simulink model "Hybrid_P2_Parallel"  (R2017b)
settings: Solver=FixedStepAuto  StartTime=0.0  StopTime=length(Speed)  FixedStep=0.01  MaxStep=0.01  RelTol=1e-3  EnableMultiTasking=on
PostLoadFcn:
  | , if any(exist('dsrtsu_mdlpostloadfcn', 'file') == [2, 3, 6]), try dsrtsu_mdlpostloadfcn('Execute', bdroot); catch fprintf('Error in PostLoadFcn (dsrtsu_mdlpostloadfcn) for model "%s":\n %s\n', bdroot, lasterr); end, end,
undefined symbols (not defined in the file): APP1_OOR, APP2_OOR, APP_Mismatch, Brk_Flt, cal, clt, Clutch, Clutch2, ClutchEngag, eng, Engine, EngOverTemp, ENGTRQ_MSMCH_Degraded_CP, ENGTRQ_MSMCH_ErrCritical_CP, ENGTRQ_MSMCH_LimpHome_CP, EngTrqMismatch, ess, ESSOverTemp, gb, KeyPos_Flt, LossCAN, MCUOverTemp, mot, MotDirMismatch, MotOverTemp, MotTrqMismatch, mph2kph, PRNDL_Flt, RegenFault, time, tloop
libraries: simulink x100, EC2_libraries x7, powerlib_meascontrol x2, lib_Actuators x1, CalculationGallon x1, lib_Chassis x1, autolibcoupling x1, autolibsharedcoupling x1, lib_DCDC x1, lib_Differential x1, lib_EMachine_2017a x1, lib_HVESS x1
(part 1 of 7)
settings Model: DSRTSU_INTERNAL_RTI_VER=480  DSRTSU_INTERNAL_RTI_TYPE=rti1006  RTICANMMDATA=struct('GeneralSetupData',struct('modelroot','D:\EcoCAR3\Controls\HIL\Y3\P2_Parallel_MIL_Model','generalsettings',struct('filesettings',struct('destfolder',struct('Name','RTICANMM_FILES','Check',1),'buildfolder',struct('Name','.','Check',1),'AbsDestfolder',struct('Name','D:\EcoCAR3\Controls\HIL\Y3\P2_Parallel_MIL_Model\RTICANMM_FILES'),'AbsBuildfolder',struct('Name','D:\EcoCAR3\Controls\HIL\Y3\P2_Parallel_MIL_Model'))),'options',struct('addpaths',1,'rmpaths',1,'addtrcexclusion',logical(1),'cannavigator',struct('checkmonitoring',0),'show_usrtrc',0,'use_usrtrc',0),'advanced',struct('options',[1 1 1 1 1 1 1 1 1 1 1 1 1 1 1 1 1 1 1 1 1 1 1 1 1 1 1 1 1 1 1 1 1 1 1 1 1 1 1 1 1 1 1 1 1 1 1 1 1 1 1 1 1 1 1 1 1 1 1 1 1 1 1 1 1 1 1 1 1 1 1 1 1 1 1 1 1 1 1 1 1 1 1 1 1 1 1 1 1 1 1 1 1 1 1 1 1 1 1 1]),'MPSetup',{{}},'modelname','P2_Parallel_MIL_02_16_2017','block','P2_Parallel_MIL_02_16_2017'))  DSRTSU_INTERNAL_RTIFPGA=70  SimulationMode=accelerator  Creator=EcoCar  LastModifiedBy=Lyu19
settings SolverCC: ExtrapolationOrder=1  NumberNewtonIterations=4
settings OptimizationCC: BlockReduction=off  OptimizeBlockIOStorage=off  BufferReuse=off  GlobalBufferReuse=off  ExpressionFolding=off  LocalBlockOutputs=off  EfficientMapNaN2IntZero=off
settings DebuggingCC: AllowSymbolicDim=off  NonBusSignalsTreatedAsBus=warning  SFUnexpectedBacktrackingDiag=warning  SFNoUnconditionalDefaultTransitionDiag=warning  SFExecutionAtInitializationDiag=none
settings HardwareCC: ProdBitPerPointer=32  ProdBitPerSizeT=32  ProdBitPerPtrDiffT=32  ProdLargestAtomicInteger=Integer  ProdWordSize=32  ProdHWDeviceType=Custom Processor->Custom  TargetBitPerPointer=64  TargetBitPerSizeT=64  TargetBitPerPtrDiffT=64  TargetLongLongMode=on  TargetIntDivRoundTo=Zero  TargetEndianess=LittleEndian  TargetWordSize=64  TargetHWDeviceType=MATLAB Host  ProdEqTarget=off
settings ModelReferenceCC: PropagateSignalLabelsOutOfModel=off
settings CodeAppCC: MaxIdLength=128  StateflowObjectComments=on
settings GRTTargetCC: TargetLangStandard=C89/C90 (ANSI)  CombineOutputUpdateFcns=off  GRTInterface=on
settings ConfigComp: CovMetricSettings=dw  CovHtmlReporting=on  CovSaveCumulativeToWorkspaceVar=on  CovSaveSingleToWorkspaceVar=on  CovExternalEMLEnable=off
settings SimscapeCC: SimscapeNormalizeSystem=off

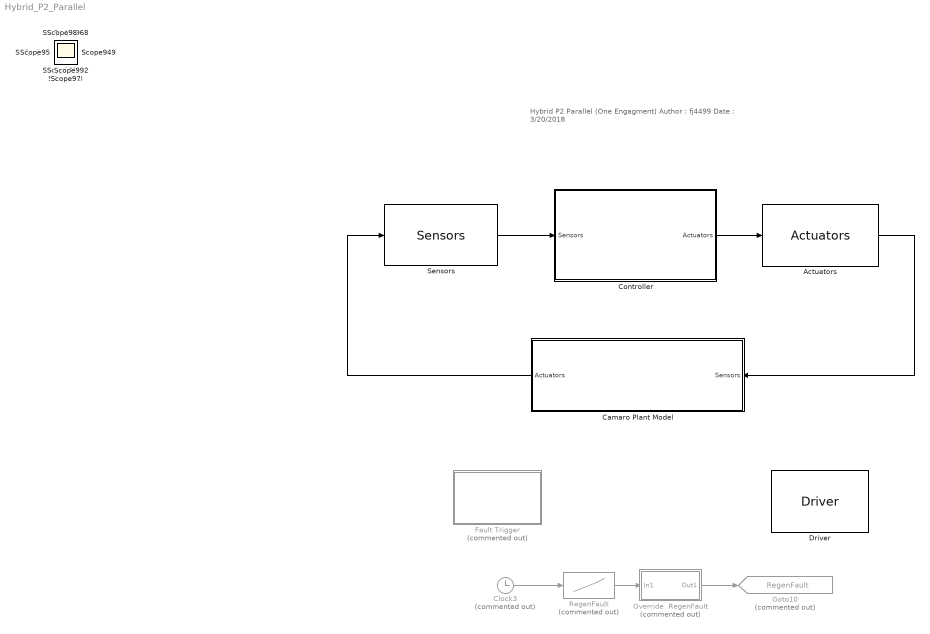
== system Hybrid_P2_Parallel ==
  note: Hybrid P2 Parallel (One Engagment)
      |
      | Author : fj4499
      | Date : 3/20/2018
  Actuators : lib_Actuators/Actuators
  Camaro Plant Model : Subsystem
      mask Display: image('Images/Vehicle.jpg')
  Clock3 : Clock  Commented=on
  Controller : Subsystem
      mask Display: image('Images/HCU.jpg')
  Driver : lib_Driver/Driver  SystemSampleTime=-1
  "Fault Trigger " : Subsystem  Commented=on  mask(Fault Trigger){Mismatch_APP_ON=on, APP1_OOR_ON=on, APP2_OOR_ON=on, Brk_Flt_ON=on, KeyPos_Flt_ON=on, PRNDL_Flt_ON=on, LossCAN_ON=on, MotTrqMismatch_ON=on, MotDirMismatch_ON=on, EngTrqMismatch_ON=on, MotOverTemp_ON=on, MCUOverTemp_ON=on, EngOverTemp_ON=on, ESSOverTemp_ON=on, ClutchEngagFlt=on}
      mask help:
      | Check the box: override the fault (Control Port value=1;)
      | Uncheck the box: Implement the fault (Control Port value=0;)
      mask DialogControl DriverInterfaceFault Prompt: Driver Interface Fault
      mask DialogControl Container3 Prompt: Component Fault
      mask Display:
      | plot([1 2 2.01 3 4], [0 0 1 1 1]);
      | disp('           Fault Trigger')
  Goto10 : Goto  Commented=on  GotoTag=RegenFault  TagVisibility=global
  Override  RegenFault : Subsystem  Commented=on
  RegenFault : Lookup  Commented=on  InputValues=time  Table=RegenFault  LookUpMeth=Interpolation-Use End Values  OutDataTypeStr=int8
  Sensors : lib_Sensors_2017a/Sensors
  Scope{,1..133} (134 alike) : Scope
  wires:
  Clock3/1 -> RegenFault/1
  RegenFault/1 -> Override  RegenFault/1(In1)
  Override  RegenFault/1(Out1) -> Goto10/1
  Controller/1(Actuators) -> Actuators/1
  Actuators/1 -> Camaro Plant Model/1(Sensors)
  Camaro Plant Model/1(Actuators) -> Sensors/1
  Sensors/1 -> Controller/1(Sensors)

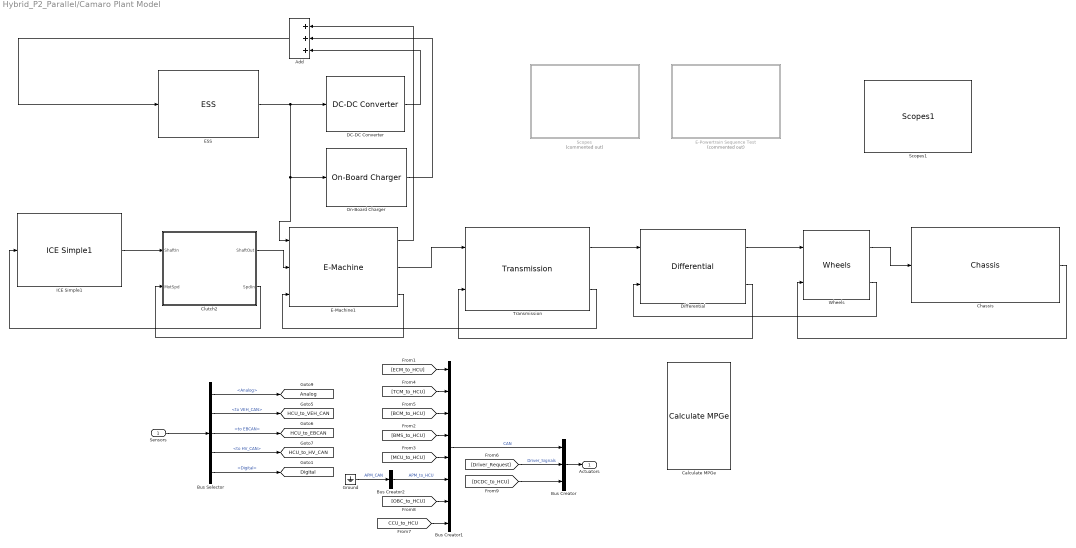
== system Hybrid_P2_Parallel/Camaro Plant Model ==
  Sensors : Inport
  Add : Sum  Inputs=+++
      mask Display:
      | port_label('input',1,'+');
      | port_label('input',2,'+');
      | port_label('input',3,'+');
  Bus Creator : BusCreator  Inputs=3
  Bus Creator1 : BusCreator  Inputs=8
  Bus Creator2 : BusCreator  Inputs=1
  Bus Selector : BusSelector  OutputSignals=Analog,CAN.to VEH_CAN,CAN.to EBCAN,CAN.to HV_CAN,Digital
  Calculate MPGe : CalculationGallon/Calculate MPGe
  Chassis : lib_Chassis/Chassis  SystemSampleTime=-1
  Clutch2 : Subsystem  AncestorBlock=Clutch/Clutch2
      mask Display:
      | image('Images/Clutch.jpg')
      | color('red');
      | port_label('Input',1,'ShaftIn');
      | port_label('Input',2,'SpdOut');
      | port_label('Output',1,'ShaftOut');
      | port_label('Output',2,'SpdIn');
  DC-DC Converter : lib_DCDC/DC-DC Converter  SystemSampleTime=-1
  Differential : lib_Differential/Differential  SystemSampleTime=-1
  E-Machine1 : lib_EMachine_2017a/E-Machine  SystemSampleTime=-1
  E-Powertrain Sequence Test : Subsystem  Commented=on
      mask Display: image('Images/Scope.jpg')
  ESS : lib_HVESS/ESS  SystemSampleTime=-1
  Ground : Ground
  ICE Simple1 : lib_Engine/ICE Simple1  SystemSampleTime=-1
  On-Board Charger : lib_OBC/On-Board Charger  SystemSampleTime=-1
      settings: SourceProductName=The database C:\Users\vrajm\AppData\Roaming\MathWorks\MATLAB\R2017b\slblocks_master.db is locked, or a table in the database is locked. (database is locked)
  Scopes : Subsystem  Commented=on
      mask Display: image('Images/Scope.jpg')
  Scopes1 : Scope_new/Scopes1  SystemSampleTime=-1
  Transmission : lib_Transmission/Transmission  SystemSampleTime=-1
  Wheels : lib_Wheels/Wheels  SystemSampleTime=-1
  Actuators : Outport
  tag scope: Analog=global, Digital=global, HCU_to_EBCAN=global, HCU_to_HV_CAN=global, HCU_to_VEH_CAN=global
  wires:
  Differential/1 -> Wheels/1
  Wheels/1 -> Chassis/1
  Chassis/1 -> Wheels/2
  Differential/2 -> Transmission/2
  Transmission/1 -> Differential/1
  ESS/1 -> E-Machine1/1, On-Board Charger/1, DC-DC Converter/1
  DC-DC Converter/1 -> Add/3
  On-Board Charger/1 -> Add/2
  Add/1 -> ESS/1
  Transmission/2 -> E-Machine1/3
  E-Machine1/2 -> Transmission/1
  E-Machine1/1 -> Add/1
  Bus Creator/1 -> Actuators/1
  Sensors/1 -> Bus Selector/1
  Bus Selector/1 -> [Analog]  "<Analog>"
  Bus Selector/2 -> [HCU_to_VEH_CAN]  "<to VEH_CAN>"
  Bus Selector/3 -> [HCU_to_EBCAN]  "<to EBCAN>"
  Bus Selector/4 -> [HCU_to_HV_CAN]  "<to HV_CAN>"
  Bus Selector/5 -> [Digital]  "<Digital>"
  Wheels/2 -> Differential/2
  E-Machine1/3 -> Clutch2/2(MotSpd)
  [ECM_to_HCU] -> Bus Creator1/1
  [TCM_to_HCU] -> Bus Creator1/2
  [BCM_to_HCU] -> Bus Creator1/3
  [BMS_to_HCU] -> Bus Creator1/4
  [MCU_to_HCU] -> Bus Creator1/5
  Bus Creator2/1 -> Bus Creator1/6  "APM_to_HCU"
  [OBC_to_HCU] -> Bus Creator1/7
  Bus Creator1/1 -> Bus Creator/1  "CAN"
  [Driver_Request] -> Bus Creator/2  "Driver_Signals"
  [DCDC_to_HCU] -> Bus Creator/3
  Ground/1 -> Bus Creator2/1  "APM_CAN"
  Clutch2/1(ShaftOut) -> E-Machine1/2
  Clutch2/2(SpdIn) -> ICE Simple1/1
  [CCU_to_HCU] -> Bus Creator1/8
  ICE Simple1/1 -> Clutch2/1(ShaftIn)

== system Hybrid_P2_Parallel/Controller ==
  Sensors : Inport
  HSC : Subsystem
  Actuators : Outport
  wires:
  HSC/1(Actuators) -> Actuators/1
  Sensors/1 -> HSC/1(Sensors)

== system Hybrid_P2_Parallel/Fault Trigger  ==
  Clock3 : Clock
  Component Diagnostics setting : Subsystem
  Driver Interface Diagnostics setting : Subsystem
  wires:
  Clock3/1 -> Component Diagnostics setting/1(time), Driver Interface Diagnostics setting/1(time)

== system Hybrid_P2_Parallel/Override  RegenFault ==
  note: This subsystem is used to override the model value of a signal to a constant value
  note: Override Switch Subsystem
  In1 : Inport
  Constant : Constant  Value=0
  Multiport Switch : MultiPortSwitch  DataPortOrder=Zero-based contiguous  Inputs=2
  Signal Override Switch 0 = Use Model 1 = Use Constant : Constant  Value=0
  Out1 : Outport
  wires:
  Signal Override Switch 0 = Use Model 1 = Use Constant/1 -> Multiport Switch/1
  In1/1 -> Multiport Switch/2
  Multiport Switch/1 -> Out1/1
  Constant/1 -> Multiport Switch/3

== system Hybrid_P2_Parallel/Camaro Plant Model/Clutch2 ==
  ShaftIn : Inport
  MotSpd : Inport  Port=2
  CCU : Subsystem
      mask Display: image('SoftECU.jpg')
  Clutch Plant : Subsystem
      mask Display:
      | image('Images/Clutch.jpg')
      | color('red');
      | port_label('Input',2,'ShaftIn');
      | port_label('Input',3,'SpdOut');
      | port_label('Output',3,'ShaftOut');
      | port_label('Output',2,'SpdIn');
  ShaftOut : Outport
  SpdIn : Outport  Port=2
  tag scope: CCU_to_HCU=global
  wires:
  Clutch Plant/1(Out1) -> CCU/2(Clutch Feedback)
  CCU/1("CCU_CAN ") -> [CCU_to_HCU]
  Clutch Plant/3(MotorShaft Out) -> ShaftOut/1
  Clutch Plant/2(Spdin) -> SpdIn/1
  MotSpd/1 -> Clutch Plant/3(SpdOut)
  ShaftIn/1 -> Clutch Plant/2(In2)
  CCU/2("Actuator command ") -> Clutch Plant/1(In1)
  [HCU_to_EBCAN] -> CCU/1(HSC Commands)

== system Hybrid_P2_Parallel/Camaro Plant Model/E-Powertrain Sequence Test ==
  Scope : Scope  NumInputPorts=4
  Terminator : Terminator
  wires:
  [KeyPosition] -> Scope/1  "Key Position"
  [InverterEnabled] -> Scope/2  "Inverter Enabled"
  [MO_BMS_Sollmodus] -> Scope/3  "Contactors Status"
  [DCDC_Status] -> Scope/4  "DCDC Status"
  [ShftLvrPos] -> Terminator/1  "Shift Lever Postion"

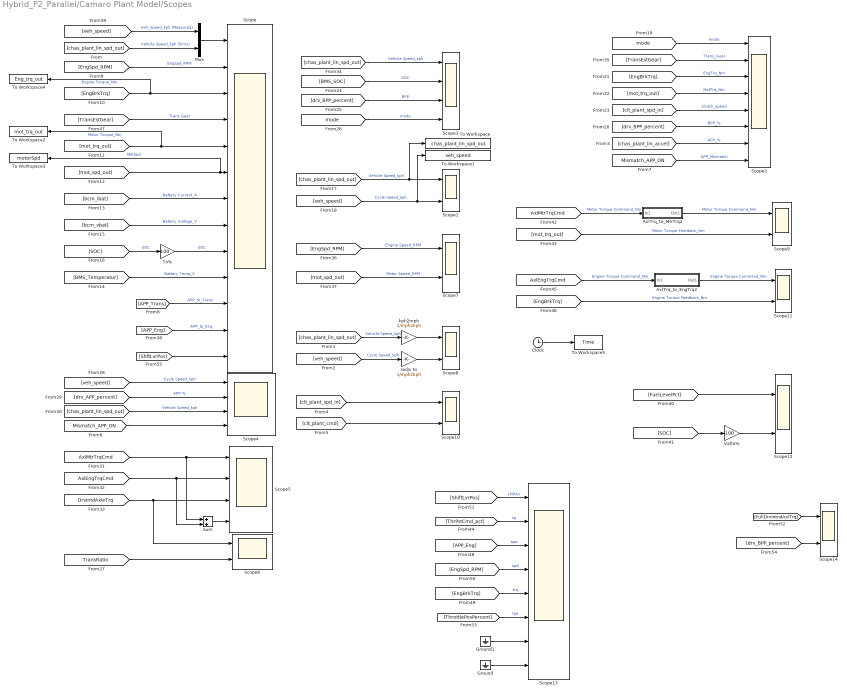
== system Hybrid_P2_Parallel/Camaro Plant Model/Scopes ==
  AxlTrq_to_EngTrq2 : Subsystem
  AxlTrq_to_MtrTrq2 : Subsystem
  Clock : Clock
      settings: Decimation=WORKSPACE_DECIMATION
  Ground : Ground
  Ground1 : Ground
  Mux : Mux  Inputs=2
  Scope : Scope  NumInputPorts=13
  Scope{1,6..12,14} (9 alike) : Scope  NumInputPorts=2
  Scope13 : Scope  NumInputPorts=8
  Scope2 : Scope  NumInputPorts=8
  Scope3 : Scope  NumInputPorts=4
  Scope4 : Scope  NumInputPorts=4
  Scope5 : Scope  NumInputPorts=4
  Sum : Sum
  To Workspace : ToWorkspace  VariableName=chas_plant_lin_spd_out  SampleTime=-1
  To Workspace1 : ToWorkspace  VariableName=veh_speed  SampleTime=-1
  To Workspace2 : ToWorkspace  VariableName=mot_trq_out  SampleTime=-1
  To Workspace3 : ToWorkspace  VariableName=motorSpd  SampleTime=-1
  To Workspace4 : ToWorkspace  VariableName=Eng_trq_out  SampleTime=-1
  To Workspace5 : ToWorkspace  VariableName=Time  SampleTime=-1
      settings: Decimation=WORKSPACE_DECIMATION
  To% : Gain  Gain=100
  Valto% : Gain  Gain=100
  kph2mph : Gain  Gain=1/mph2kph
  "rad/s to " : Gain  Gain=1/mph2kph
  wires:
  [chas_plant_lin_spd_out] -> Mux/2  "Vehicle Speed_kph (Simu)"
  [EngSpd_RPM] -> Scope/2  "EngSpd_RPM"
  [EngBrkTrq] -> To Workspace4/1, Scope/3  "Engine Torque_Nm"
  [mot_spd_out] -> To Workspace3/1, Scope/6  "MotSpd"
  [BMS_Temperatur] -> Scope/10  "Battery Temp_C"
  [mot_trq_out] -> To Workspace2/1, Scope/5  "Motor Torque_Nm"
  To%/1 -> Scope/9  "SOC"
  [TransEstGear] -> Scope/4  "Trans Gear"
  [bcm_ibat] -> Scope/7  "Battery Current_A"
  [chas_plant_lin_spd_out] -> Scope3/1  "Vehicle Speed_kph"
  [BMS_SOC] -> Scope3/2  "SOC"
  [drv_BPP_percent] -> Scope3/3  "BPP"
  [mode] -> Scope3/4  "mode"
  [chas_plant_lin_spd_out] -> To Workspace/1, Scope1/1  "Vehicle Speed_kph"
  [veh_speed] -> To Workspace1/1, Scope1/2  "Cycle Speed_kph"
  [mode] -> Scope2/1  "mode"
  [EngBrkTrq] -> Scope2/3  "EngTrq_Nm"
  [mot_trq_out] -> Scope2/4  "MotTrq_Nm"
  [clt_plant_spd_in] -> Scope2/5  "Clutch_speed"
  [EngSpd_RPM] -> Scope7/1  "Engine Speed_RPM"
  [mot_spd_out] -> Scope7/2  "Motor Speed_RPM"
  [veh_speed] -> Scope4/1  "Cycle Speed_kph"
  [drv_APP_percent] -> Scope4/2  "APP %"
  [chas_plant_lin_spd_out] -> Scope4/3  "Vehicle Speed_kph"
  [AxlMtrTrqCmd] -> Sum/1, Scope5/1
  [AxlEngTrqCmd] -> Sum/2, Scope5/2
  [DrvIntdAxleTrq] -> Scope6/1, Scope5/3
  Sum/1 -> Scope5/4
  [TransRatio] -> Scope6/2
  [AxlMtrTrqCmd] -> AxlTrq_to_MtrTrq2/1(In1)  "Motor Torque Command_Nm"
  [mot_trq_out] -> Scope9/2  "Motor Torque Feedback_Nm"
  [AxlEngTrqCmd] -> AxlTrq_to_EngTrq2/1(In1)  "Engine Torque Command_Nm"
  [EngBrkTrq] -> Scope11/2  "Engine Torque Feedback_Nm"
  [chas_plant_lin_spd_out] -> kph2mph/1  "Vehicle Speed_kph"
  [veh_speed] -> "rad/s to "/1  "Cycle Speed_kph"
  kph2mph/1 -> Scope8/1
  "rad/s to "/1 -> Scope8/2
  [TransEstGear] -> Scope2/2  "Trans_Gear"
  [drv_BPP_percent] -> Scope2/6  "BPP_%"
  [chas_plant_lin_accel] -> Scope2/7  "APP_%"
  AxlTrq_to_MtrTrq2/1(Out1) -> Scope9/1  "Motor Torque Command_Nm"
  AxlTrq_to_EngTrq2/1(Out1) -> Scope11/1  "Engine Torque Command_Nm"
  [bcm_vbat] -> Scope/8  "Battery Voltage_V"
  [clt_plant_spd_in] -> Scope10/1
  [clt_plant_cmd] -> Scope10/2
  [Mismatch_APP_ON] -> Scope4/4
  [Mismatch_APP_ON] -> Scope2/8  "APP_Mismatch"
  [SOC] -> To%/1  "SOC"
  [APP_Trans] -> Scope/11  "APP_to_Trans"
  [APP_Eng] -> Scope/12  "APP_to_Eng"
  Mux/1 -> Scope/1
  [veh_speed] -> Mux/1  "Veh_Speed_kph (Measured)"
  Clock/1 -> To Workspace5/1
  [FuelLevelPct] -> Scope12/1
  [SOC] -> Valto%/1
  Valto%/1 -> Scope12/2
  [ShiftLvrPos] -> Scope13/1  "shiftlvr"
  [ThrPstCmd_pct] -> Scope13/2  "tp"
  [APP_Eng] -> Scope13/3  "app"
  [EngSpd_RPM] -> Scope13/4  "spd"
  [EngBrkTrq] -> Scope13/5  "trq"
  [ThrottlePosPercent] -> Scope13/6  "tpp"
  Ground/1 -> Scope13/8
  Ground1/1 -> Scope13/7
  [FullDrvIntndAxlTrq] -> Scope14/1
  [drv_BPP_percent] -> Scope14/2
  [ShftLvrPos] -> Scope/13

== system Hybrid_P2_Parallel/Controller/HSC ==
  Sensors : Inport
  Camaro Fault Detection : Subsystem
  Driver_Requests : Subsystem  RequirementInfo={} %GIDa_7669cec5_5f7d_402f_871c_1fc3f99e6295
  Powertrain Manager : Subsystem
  Actuators : Outport
  wires:
  Driver_Requests/1(DriverRequests) -> Powertrain Manager/2(Driver Request)
  Camaro Fault Detection/1(Diagnostic) -> Driver_Requests/2("Diagnostic "), Powertrain Manager/3(Fault Detection)
  Powertrain Manager/1(Out1) -> Actuators/1
  Sensors/1 -> Driver_Requests/1(Sensors), Powertrain Manager/1(Sensors), Camaro Fault Detection/1(Sensors)
  Powertrain Manager/2(Controls) -> Driver_Requests/3("Controls ")

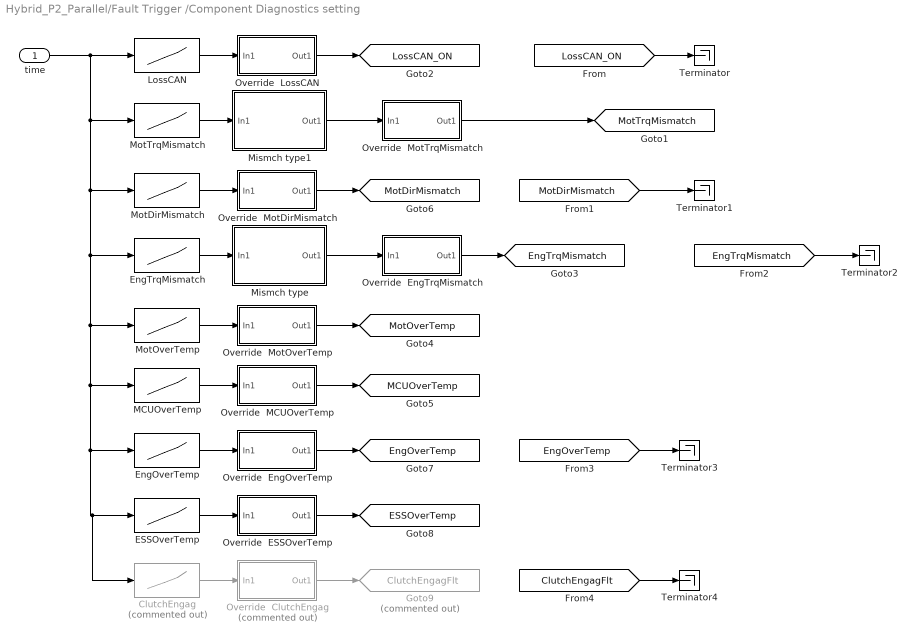
== system Hybrid_P2_Parallel/Fault Trigger /Component Diagnostics setting ==
  time : Inport
  ClutchEngag : Lookup  Commented=on  InputValues=time  Table=ClutchEngag  LookUpMeth=Interpolation-Use End Values  OutDataTypeStr=int8
  ESSOverTemp : Lookup  InputValues=time  Table=ESSOverTemp  LookUpMeth=Interpolation-Use End Values  OutDataTypeStr=int8
  EngOverTemp : Lookup  InputValues=time  Table=EngOverTemp  LookUpMeth=Interpolation-Use End Values  OutDataTypeStr=int8
  EngTrqMismatch : Lookup  InputValues=time  Table=EngTrqMismatch  LookUpMeth=Interpolation-Use End Values  OutDataTypeStr=int8
  Goto9 : Goto  Commented=on  GotoTag=ClutchEngagFlt  TagVisibility=global
  LossCAN : Lookup  InputValues=time  Table=LossCAN  LookUpMeth=Interpolation-Use End Values  OutDataTypeStr=int8
  MCUOverTemp : Lookup  InputValues=time  Table=MCUOverTemp  LookUpMeth=Interpolation-Use End Values  OutDataTypeStr=int8
  Mismch type : Subsystem
  Mismch type1 : Subsystem
  MotDirMismatch : Lookup  InputValues=time  Table=MotDirMismatch  LookUpMeth=Interpolation-Use End Values  OutDataTypeStr=int8
  MotOverTemp : Lookup  InputValues=time  Table=MotOverTemp  LookUpMeth=Interpolation-Use End Values  OutDataTypeStr=int8
  MotTrqMismatch : Lookup  InputValues=time  Table=MotTrqMismatch  LookUpMeth=Interpolation-Use End Values  OutDataTypeStr=int8
  Override  ClutchEngag : Subsystem  Commented=on
  Override  ESSOverTemp : Subsystem
  Override  EngOverTemp : Subsystem
  Override  EngTrqMismatch : Subsystem
  Override  LossCAN : Subsystem
  Override  MCUOverTemp : Subsystem
  Override  MotDirMismatch : Subsystem
  Override  MotOverTemp : Subsystem
  Override  MotTrqMismatch : Subsystem
  Terminator{,1..4} (5 alike) : Terminator
  tag scope: ESSOverTemp=global, EngOverTemp=global, EngTrqMismatch=global, LossCAN_ON=global, MCUOverTemp=global, MotDirMismatch=global, MotOverTemp=global, MotTrqMismatch=global
  wires:
  MotOverTemp/1 -> Override  MotOverTemp/1(In1)
  LossCAN/1 -> Override  LossCAN/1(In1)
  time/1 -> LossCAN/1, MotTrqMismatch/1, EngTrqMismatch/1, MotOverTemp/1, MCUOverTemp/1, EngOverTemp/1, ClutchEngag/1, ESSOverTemp/1, MotDirMismatch/1
  Override  LossCAN/1(Out1) -> [LossCAN_ON]
  Override  MCUOverTemp/1(Out1) -> [MCUOverTemp]
  Override  EngTrqMismatch/1(Out1) -> [EngTrqMismatch]
  Override  MotDirMismatch/1(Out1) -> [MotDirMismatch]
  MotDirMismatch/1 -> Override  MotDirMismatch/1(In1)
  Override  MotTrqMismatch/1(Out1) -> [MotTrqMismatch]
  MotTrqMismatch/1 -> Mismch type1/1(In1)
  EngTrqMismatch/1 -> Mismch type/1(In1)
  Override  MotOverTemp/1(Out1) -> [MotOverTemp]
  MCUOverTemp/1 -> Override  MCUOverTemp/1(In1)
  Override  EngOverTemp/1(Out1) -> [EngOverTemp]
  EngOverTemp/1 -> Override  EngOverTemp/1(In1)
  Override  ESSOverTemp/1(Out1) -> [ESSOverTemp]
  ESSOverTemp/1 -> Override  ESSOverTemp/1(In1)
  Override  ClutchEngag/1(Out1) -> Goto9/1
  ClutchEngag/1 -> Override  ClutchEngag/1(In1)
  Mismch type/1(Out1) -> Override  EngTrqMismatch/1(In1)
  Mismch type1/1(Out1) -> Override  MotTrqMismatch/1(In1)
  [LossCAN_ON] -> Terminator/1
  [MotDirMismatch] -> Terminator1/1
  [EngTrqMismatch] -> Terminator2/1
  [EngOverTemp] -> Terminator3/1
  [ClutchEngagFlt] -> Terminator4/1

== system Hybrid_P2_Parallel/Fault Trigger /Driver Interface Diagnostics setting ==
  time : Inport
  APP1_OOR : Lookup  InputValues=time  Table=APP1_OOR  LookUpMeth=Interpolation-Use End Values  OutDataTypeStr=int8
  APP2_OOR : Lookup  InputValues=time  Table=APP2_OOR  LookUpMeth=Interpolation-Use End Values  OutDataTypeStr=int8
  APP_Mismatch : Lookup  InputValues=time  Table=APP_Mismatch  LookUpMeth=Interpolation-Use End Values  OutDataTypeStr=int8
  BPP_Flt : Lookup  InputValues=time  Table=Brk_Flt  LookUpMeth=Interpolation-Use End Values  OutDataTypeStr=int8
  KeyPos_Flt : Lookup  InputValues=time  Table=KeyPos_Flt  LookUpMeth=Interpolation-Use End Values  OutDataTypeStr=int8
  Override  APP1_OOR : Subsystem
  Override  APP2_OOR : Subsystem
  Override  APP_Mismatch : Subsystem
  Override  BPP_Flt : Subsystem
  Override  KeyPos_Flt : Subsystem
  Override  PRNDL_Flt : Subsystem
  PRNDL_Flt : Lookup  InputValues=time  Table=PRNDL_Flt  LookUpMeth=Interpolation-Use End Values  OutDataTypeStr=int8
  Terminator : Terminator
  Terminator1 : Terminator
  tag scope: APP1_OOR_ON=global, APP2_OOR_ON=global, Brk_Flt=global, KeyPos_Flt_ON=global, Mismatch_APP_ON=global, PRNDL_Flt_ON=global
  wires:
  PRNDL_Flt/1 -> Override  PRNDL_Flt/1(In1)
  Override  KeyPos_Flt/1(Out1) -> [KeyPos_Flt_ON]
  BPP_Flt/1 -> Override  BPP_Flt/1(In1)
  APP1_OOR/1 -> Override  APP1_OOR/1(In1)
  Override  APP1_OOR/1(Out1) -> [APP1_OOR_ON]
  APP2_OOR/1 -> Override  APP2_OOR/1(In1)
  Override  APP2_OOR/1(Out1) -> [APP2_OOR_ON]
  Override  BPP_Flt/1(Out1) -> [Brk_Flt]
  Override  PRNDL_Flt/1(Out1) -> [PRNDL_Flt_ON]
  time/1 -> APP_Mismatch/1, APP2_OOR/1, PRNDL_Flt/1, KeyPos_Flt/1, BPP_Flt/1, APP1_OOR/1
  KeyPos_Flt/1 -> Override  KeyPos_Flt/1(In1)
  Override  APP_Mismatch/1(Out1) -> [Mismatch_APP_ON]  "APP_Mismatch"
  APP_Mismatch/1 -> Override  APP_Mismatch/1(In1)
  [APP1_OOR_ON] -> Terminator/1
  [PRNDL_Flt_ON] -> Terminator1/1

== system Hybrid_P2_Parallel/Camaro Plant Model/Clutch2/CCU ==
  HSC Commands : Inport
  Clutch Feedback : Inport  Port=2
  Bus Creator : BusCreator  Inputs=4
  Bus Creator1 : BusCreator  Inputs=1
  Bus Selector : BusSelector  OutputSignals=MY15_CCU_posDes,MY15_CCU_stModeReq
  Bus Selector1 : BusSelector  OutputSignals=CY01_pCurr
  Counter Free-Running : simulink/Sources/Counter Free-Running  NumBits=15  tsamp=-1
  Data Type Conversion : DataTypeConversion
  Data Type Conversion1 : DataTypeConversion
  "CCU_CAN " : Outport
  "Actuator command " : Outport  Port=2
  wires:
  Clutch Feedback/1 -> Bus Selector1/1
  Data Type Conversion1/1 -> Bus Creator/2  "CY01_stMode"
  Bus Selector/2 -> Data Type Conversion1/1  "<MY15_CCU_stModeReq>"
  Counter Free-Running/1 -> Bus Creator/3  "CY01_Counter"
  Bus Creator1/1 -> "Actuator command "/1
  Bus Creator/1 -> "CCU_CAN "/1  "CCU_CAN"
  Data Type Conversion/1 -> Bus Creator/1, Bus Creator1/1  "CY01_posCurr"
  Bus Selector/1 -> Data Type Conversion/1  "<MY15_CCU_posDes>"
  HSC Commands/1 -> Bus Selector/1
  Bus Selector1/1 -> Bus Creator/4  "<CY01_pCurr>"

== system Hybrid_P2_Parallel/Camaro Plant Model/Clutch2/Clutch Plant ==
  In1 : Inport
  In2 : Inport  Port=2
  SpdOut : Inport  Port=3
  " Actuator" : Subsystem
  " Sensors " : Subsystem
  Bus Creator1 : BusCreator  Inputs=2
  Bus Selector : BusSelector  OutputSignals=eng_trq_out_Nm
  Bus Selector1 : BusSelector  OutputSignals=eng_inertia_out
  Clutch : autolibcoupling/Disc Clutch  port_config=Simulink  Reff=0.121  Ndisk=1  Aeff=0.02129  Jin=Engine.Inertia + (0.75*clt.plant.init.inertia)  Jout=.1 + (0.25*clt.plant.init.inertia)  muk=0.25  mus=0.3  bin=.001*2  bout=.001*2  win_o=0  wout_o=0  tauC=0.01*10  InitiallyLocked=on  maxAbsSpd=3000  blkID=1
      settings: SourceProductName=Powertrain Blockset  SourceProductBaseCode=PW
  Driveshaft Compliance1 : autolibsharedcoupling/Torsional Compliance  port_config=Two-way connection  k=1000000  b=100  theta_o=0  domega_o=0  omega_c=100  blkID=0
      settings: SourceProductName=Powertrain Blockset
  In4 : InportShadow
  Memory : Memory
  Subsystem : Subsystem
  Terminator : Terminator
  Two-Way Connection2 : TwoWayConnection
  Two-Way Connection3 : TwoWayConnection
  Out1 : Outport
  Spdin : Outport  Port=2
  MotorShaft Out : Outport  Port=3
  tag scope: CltEngPressCmd=global
  wires:
  " Sensors "/1(Pressure) -> Out1/1
  In4/1 -> " Sensors "/1(In1)
  Bus Selector/1 -> Clutch/2  "<eng_trq_out_Nm>"
  [CltEngPressCmd] -> Clutch/1
  " Actuator"/1(Clutch Engagement Pressure Command) -> [CltEngPressCmd]
  Clutch/1 -> Terminator/1
  In1/1 -> " Actuator"/1(In1)
  Clutch/3 -> Two-Way Connection2/1
  SpdOut/1 -> Two-Way Connection3/1
  In2/1 -> Bus Selector1/1, Bus Selector/1
  Memory/1 -> Spdin/1
  Two-Way Connection2/1 -> Clutch/3
  Two-Way Connection3/1 -> Bus Creator1/1  "Motor Torque In"
  Clutch/2 -> Memory/1
  [CltEngPressCmd] -> Subsystem/2(Clutch Engagement Pressure)
  Bus Selector1/1 -> Subsystem/1(Engine Inertia Out)  "<eng_inertia_out>"
  Bus Creator1/1 -> MotorShaft Out/1
  Subsystem/1(Motor Inertia In) -> Bus Creator1/2  "Motor Inertia In"
  connections:
  Driveshaft Compliance1/LConn1 -- Two-Way Connection2/RConn1
  Two-Way Connection3/RConn1 -- Driveshaft Compliance1/RConn1

== system Hybrid_P2_Parallel/Camaro Plant Model/Scopes/AxlTrq_to_EngTrq2 ==
  note: //From engine axle torque to engine torque//
  In1 : Inport
  Compare To Constant : simulink/Logic and Bit Operations/Compare To Constant  relop===  const=0  OutDataTypeStr=boolean
  Constant1 : Constant  Value=max(gb.plant.init.ratio.map)
  Constant5 : Constant  Value=fd.plant.init.ratio
  Divide1 : Product  Inputs=*//
  Rate Limiter : RateLimiter  RisingSlewLimit=Engine.trq_uprate  FallingSlewLimit=Engine.trq_derate
  Ratio Filter : Subsystem
  Switch : Switch  Criteria=u2 > Threshold
  Out1 : Outport
  wires:
  In1/1 -> Divide1/1
  Constant5/1 -> Divide1/2
  Divide1/1 -> Rate Limiter/1
  [TransRatio] -> Ratio Filter/1(Ratio)
  Compare To Constant/1 -> Switch/2
  Constant1/1 -> Switch/1
  Switch/1 -> Divide1/3
  Rate Limiter/1 -> Out1/1
  Ratio Filter/1(Filtered_Ratio) -> Switch/3, Compare To Constant/1

== system Hybrid_P2_Parallel/Camaro Plant Model/Scopes/AxlTrq_to_MtrTrq2 ==
  note: //From motor axle torque to motor torque//
  In1 : Inport
  Compare To Constant : simulink/Logic and Bit Operations/Compare To Constant  relop===  const=0  OutDataTypeStr=boolean
  Constant1 : Constant  Value=max(gb.plant.init.ratio.map)
  Constant5 : Constant  Value=fd.plant.init.ratio
  Divide : Product  Inputs=*//
  Rate Limiter : RateLimiter  RisingSlewLimit=mcu.plant.init.trq_uprate  FallingSlewLimit=mcu.plant.init.trq_derate
  Ratio Filter : Subsystem
  Switch : Switch  Criteria=u2 > Threshold
  Out1 : Outport
  wires:
  In1/1 -> Divide/1
  Constant5/1 -> Divide/2
  Divide/1 -> Rate Limiter/1
  [TransRatio] -> Ratio Filter/1(Ratio)
  Compare To Constant/1 -> Switch/2
  Constant1/1 -> Switch/1
  Rate Limiter/1 -> Out1/1
  Switch/1 -> Divide/3
  Ratio Filter/1(Filtered_Ratio) -> Switch/3, Compare To Constant/1

== system Hybrid_P2_Parallel/Controller/HSC/Camaro Fault Detection ==
  Sensors : Inport
  Component Diagnostic : Subsystem
  Input Conversions : Subsystem
  Signal Diagnostic : Subsystem
  SystemDiag : lib_SystemDiag/SystemDiag
  Diagnostic : Outport
  wires:
  SystemDiag/1 -> Diagnostic/1
  Sensors/1 -> Input Conversions/1(RawSig)
  Input Conversions/1(VehSig) -> Signal Diagnostic/1(VehSig)
  Component Diagnostic/1(CompDiag) -> SystemDiag/1
  Signal Diagnostic/1(SignalDiag) -> Component Diagnostic/1(SignalDiag)

== system Hybrid_P2_Parallel/Controller/HSC/Driver_Requests ==
  note: Driver management
  Sensors : Inport
  "Diagnostic " : Inport  Port=2
  "Controls " : Inport  Port=3
  APP_BPP to DrvIntndAxlTrq2 : Subsystem
  DriverRequests : Outport
  wires:
  Sensors/1 -> APP_BPP to DrvIntndAxlTrq2/1(Sensors)
  APP_BPP to DrvIntndAxlTrq2/1(IntndAxlTrq) -> DriverRequests/1
  "Diagnostic "/1 -> APP_BPP to DrvIntndAxlTrq2/2(Diag)
  "Controls "/1 -> APP_BPP to DrvIntndAxlTrq2/3(Controls)

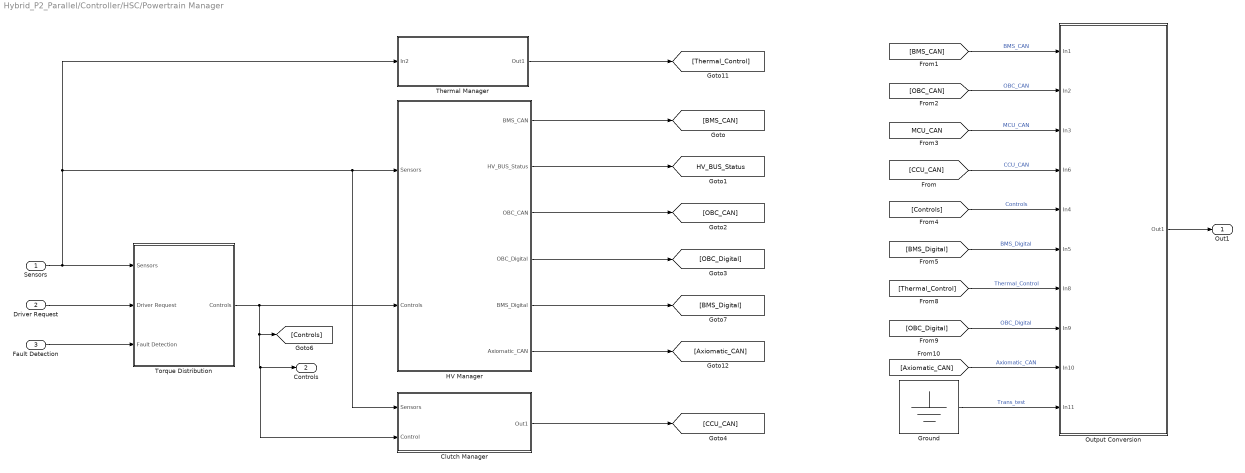
== system Hybrid_P2_Parallel/Controller/HSC/Powertrain Manager ==
  Sensors : Inport
  Driver Request : Inport  Port=2
  Fault Detection : Inport  Port=3
  Clutch Manager : Subsystem
  Ground : Ground
  HV Manager : Subsystem  AncestorBlock=lib_HVManager_PostIMG_2017a/HV Manager
  Output Conversion : Subsystem
  Thermal Manager : Subsystem  AncestorBlock=lib_ThermalManager/Thermal Manager
  Torque Distribution : Subsystem  AncestorBlock=lib_TorqueDistribution_2017a/Torque Distribution
  Out1 : Outport
  Controls : Outport  Port=2
  tag scope: HV_BUS_Status=global
  wires:
  [Thermal_Control] -> Output Conversion/7(In8)  "Thermal_Control"
  [OBC_Digital] -> Output Conversion/8(In9)  "OBC_Digital"
  [Axiomatic_CAN] -> Output Conversion/9(In10)  "Axiomatic_CAN"
  HV Manager/6(Axiomatic_CAN) -> [Axiomatic_CAN]
  Thermal Manager/1(Out1) -> [Thermal_Control]
  Fault Detection/1 -> Torque Distribution/3(Fault Detection)
  [BMS_Digital] -> Output Conversion/6(In5)  "BMS_Digital"
  HV Manager/5(BMS_Digital) -> [BMS_Digital]
  Output Conversion/1(Out1) -> Out1/1
  [Controls] -> Output Conversion/5(In4)  "Controls"
  [MCU_CAN] -> Output Conversion/3(In3)  "MCU_CAN"
  [OBC_CAN] -> Output Conversion/2(In2)  "OBC_CAN"
  [BMS_CAN] -> Output Conversion/1(In1)  "BMS_CAN"
  Driver Request/1 -> Torque Distribution/2(Driver Request)
  HV Manager/3(OBC_CAN) -> [OBC_CAN]
  HV Manager/4(OBC_Digital) -> [OBC_Digital]
  HV Manager/2(HV_BUS_Status) -> [HV_BUS_Status]
  HV Manager/1(BMS_CAN) -> [BMS_CAN]
  Ground/1 -> Output Conversion/10(In11)  "Trans_test"
  Clutch Manager/1(Out1) -> [CCU_CAN]
  Torque Distribution/1(Controls) -> HV Manager/2(Controls), Clutch Manager/2(Control), Controls/1, [Controls]
  Sensors/1 -> Clutch Manager/1(Sensors), HV Manager/1(Sensors), Thermal Manager/1(In2), Torque Distribution/1(Sensors)
  [CCU_CAN] -> Output Conversion/4(In6)  "CCU_CAN"

== system Hybrid_P2_Parallel/Fault Trigger /Component Diagnostics setting/Mismch type ==
  In1 : Inport
  Constant : Constant  Value=cal.ENGTRQ_MSMCH.Degraded_CP+1
  Constant1 : Constant  Value=cal.ENGTRQ_MSMCH.LimpHome_CP+1
  Constant2 : Constant  Value=cal.ENGTRQ_MSMCH.ErrCritical_CP+1
  Constant3 : Constant  Value=0
  Multiport Switch : MultiPortSwitch  DataPortOrder=Zero-based contiguous  Inputs=4
  Out1 : Outport
  wires:
  Constant1/1 -> Multiport Switch/4
  Constant2/1 -> Multiport Switch/5
  In1/1 -> Multiport Switch/1
  Multiport Switch/1 -> Out1/1
  Constant3/1 -> Multiport Switch/2
  Constant/1 -> Multiport Switch/3

== system Hybrid_P2_Parallel/Fault Trigger /Component Diagnostics setting/Mismch type1 ==
  In1 : Inport
  Constant : Constant  Value=cal.MOTTRQ_MSMCH.Degraded_CP+1
  Constant1 : Constant  Value=cal.MOTTRQ_MSMCH.LimpHome_CP+1
  Constant2 : Constant  Value=cal.ENGTRQ_MSMCH.ErrCritical_CP+1
  Constant3 : Constant  Value=0
  Multiport Switch : MultiPortSwitch  DataPortOrder=Zero-based contiguous  Inputs=4
  Out1 : Outport
  wires:
  Constant/1 -> Multiport Switch/3
  Constant3/1 -> Multiport Switch/2
  Multiport Switch/1 -> Out1/1
  In1/1 -> Multiport Switch/1
  Constant2/1 -> Multiport Switch/5
  Constant1/1 -> Multiport Switch/4

== system Hybrid_P2_Parallel/Fault Trigger /Component Diagnostics setting/Override  ClutchEngag ==
  note: Override Switch Subsystem
  note: This subsystem is used to override the model value of a signal to a constant value
  In1 : Inport
  Constant : Constant  Value=0
  Multiport Switch : MultiPortSwitch  DataPortOrder=Zero-based contiguous  Inputs=2
  Signal Override Switch 0 = Use Model 1 = Use Constant : Constant  Value=ClutchEngagFlt
  Out1 : Outport
  wires:
  Constant/1 -> Multiport Switch/3
  Multiport Switch/1 -> Out1/1
  In1/1 -> Multiport Switch/2
  Signal Override Switch 0 = Use Model 1 = Use Constant/1 -> Multiport Switch/1

== system Hybrid_P2_Parallel/Fault Trigger /Component Diagnostics setting/Override  ESSOverTemp ==
  note: This subsystem is used to override the model value of a signal to a constant value
  note: Override Switch Subsystem
  In1 : Inport
  Constant : Constant  Value=0
  Multiport Switch : MultiPortSwitch  DataPortOrder=Zero-based contiguous  Inputs=2
  Signal Override Switch 0 = Use Model 1 = Use Constant : Constant  Value=ESSOverTemp_ON
  Out1 : Outport
  wires:
  Signal Override Switch 0 = Use Model 1 = Use Constant/1 -> Multiport Switch/1
  In1/1 -> Multiport Switch/2
  Multiport Switch/1 -> Out1/1
  Constant/1 -> Multiport Switch/3

== system Hybrid_P2_Parallel/Fault Trigger /Component Diagnostics setting/Override  EngOverTemp ==
  note: Override Switch Subsystem
  note: This subsystem is used to override the model value of a signal to a constant value
  In1 : Inport
  Constant : Constant  Value=0
  Multiport Switch : MultiPortSwitch  DataPortOrder=Zero-based contiguous  Inputs=2
  Signal Override Switch 0 = Use Model 1 = Use Constant : Constant  Value=EngOverTemp_ON
  Out1 : Outport
  wires:
  Constant/1 -> Multiport Switch/3
  Multiport Switch/1 -> Out1/1
  In1/1 -> Multiport Switch/2
  Signal Override Switch 0 = Use Model 1 = Use Constant/1 -> Multiport Switch/1

== system Hybrid_P2_Parallel/Fault Trigger /Component Diagnostics setting/Override  EngTrqMismatch ==
  note: This subsystem is used to override the model value of a signal to a constant value
  note: Override Switch Subsystem
  In1 : Inport
  Constant : Constant  Value=0
  Multiport Switch : MultiPortSwitch  DataPortOrder=Zero-based contiguous  Inputs=2
  Signal Override Switch 0 = Use Model 1 = Use Constant : Constant  Value=EngTrqMismatch_ON
  Out1 : Outport
  wires:
  Signal Override Switch 0 = Use Model 1 = Use Constant/1 -> Multiport Switch/1
  In1/1 -> Multiport Switch/2
  Multiport Switch/1 -> Out1/1
  Constant/1 -> Multiport Switch/3

== system Hybrid_P2_Parallel/Fault Trigger /Component Diagnostics setting/Override  LossCAN ==
  note: Override Switch Subsystem
  note: This subsystem is used to override the model value of a signal to a constant value
  In1 : Inport
  Constant : Constant  Value=0
  Multiport Switch : MultiPortSwitch  DataPortOrder=Zero-based contiguous  Inputs=2
  Signal Override Switch 0 = Use Model 1 = Use Constant : Constant  Value=LossCAN_ON
  Out1 : Outport
  wires:
  Constant/1 -> Multiport Switch/3
  Multiport Switch/1 -> Out1/1
  In1/1 -> Multiport Switch/2
  Signal Override Switch 0 = Use Model 1 = Use Constant/1 -> Multiport Switch/1

== system Hybrid_P2_Parallel/Fault Trigger /Component Diagnostics setting/Override  MCUOverTemp ==
  note: This subsystem is used to override the model value of a signal to a constant value
  note: Override Switch Subsystem
  In1 : Inport
  Constant : Constant  Value=0
  Multiport Switch : MultiPortSwitch  DataPortOrder=Zero-based contiguous  Inputs=2
  Signal Override Switch 0 = Use Model 1 = Use Constant : Constant  Value=MCUOverTemp_ON
  Out1 : Outport
  wires:
  Signal Override Switch 0 = Use Model 1 = Use Constant/1 -> Multiport Switch/1
  In1/1 -> Multiport Switch/2
  Multiport Switch/1 -> Out1/1
  Constant/1 -> Multiport Switch/3

== system Hybrid_P2_Parallel/Fault Trigger /Component Diagnostics setting/Override  MotDirMismatch ==
  note: Override Switch Subsystem
  note: This subsystem is used to override the model value of a signal to a constant value
  In1 : Inport
  Constant : Constant  Value=0
  Multiport Switch : MultiPortSwitch  DataPortOrder=Zero-based contiguous  Inputs=2
  Signal Override Switch 0 = Use Model 1 = Use Constant : Constant  Value=MotDirMismatch_ON
  Out1 : Outport
  wires:
  Constant/1 -> Multiport Switch/3
  Multiport Switch/1 -> Out1/1
  In1/1 -> Multiport Switch/2
  Signal Override Switch 0 = Use Model 1 = Use Constant/1 -> Multiport Switch/1

== system Hybrid_P2_Parallel/Fault Trigger /Component Diagnostics setting/Override  MotOverTemp ==
  note: Override Switch Subsystem
  note: This subsystem is used to override the model value of a signal to a constant value
  In1 : Inport
  Constant : Constant  Value=0
  Multiport Switch : MultiPortSwitch  DataPortOrder=Zero-based contiguous  Inputs=2
  Signal Override Switch 0 = Use Model 1 = Use Constant : Constant  Value=MotOverTemp_ON
  Out1 : Outport
  wires:
  Constant/1 -> Multiport Switch/3
  Multiport Switch/1 -> Out1/1
  In1/1 -> Multiport Switch/2
  Signal Override Switch 0 = Use Model 1 = Use Constant/1 -> Multiport Switch/1

== system Hybrid_P2_Parallel/Fault Trigger /Component Diagnostics setting/Override  MotTrqMismatch ==
  note: This subsystem is used to override the model value of a signal to a constant value
  note: Override Switch Subsystem
  In1 : Inport
  Constant : Constant  Value=0
  Multiport Switch : MultiPortSwitch  DataPortOrder=Zero-based contiguous  Inputs=2
  Signal Override Switch 0 = Use Model 1 = Use Constant : Constant  Value=MotTrqMismatch_ON
  Out1 : Outport
  wires:
  Signal Override Switch 0 = Use Model 1 = Use Constant/1 -> Multiport Switch/1
  In1/1 -> Multiport Switch/2
  Multiport Switch/1 -> Out1/1
  Constant/1 -> Multiport Switch/3

== system Hybrid_P2_Parallel/Fault Trigger /Driver Interface Diagnostics setting/Override  APP1_OOR ==
  note: Signal Override Switch
      | 0 = Use Model
      | 1 = Use Constant
  note: Override Switch Subsystem
  note: This subsystem is used to override the model value of a signal to a constant value
  In1 : Inport
  APP1_OOR_ON : Constant  Value=APP1_OOR_ON
  Constant : Constant  Value=0
  Multiport Switch : MultiPortSwitch  DataPortOrder=Zero-based contiguous  Inputs=2
  Out1 : Outport
  wires:
  Constant/1 -> Multiport Switch/3
  Multiport Switch/1 -> Out1/1
  In1/1 -> Multiport Switch/2
  APP1_OOR_ON/1 -> Multiport Switch/1

== system Hybrid_P2_Parallel/Fault Trigger /Driver Interface Diagnostics setting/Override  APP2_OOR ==
  note: Signal Override Switch
      | 0 = Use Model
      | 1 = Use Constant
  note: This subsystem is used to override the model value of a signal to a constant value
  note: Override Switch Subsystem
  In1 : Inport
  APP2_OOR_ON : Constant  Value=APP2_OOR_ON
  Constant : Constant  Value=0
  Multiport Switch : MultiPortSwitch  DataPortOrder=Zero-based contiguous  Inputs=2
  Out1 : Outport
  wires:
  APP2_OOR_ON/1 -> Multiport Switch/1
  In1/1 -> Multiport Switch/2
  Multiport Switch/1 -> Out1/1
  Constant/1 -> Multiport Switch/3

== system Hybrid_P2_Parallel/Fault Trigger /Driver Interface Diagnostics setting/Override  APP_Mismatch ==
  note: Signal Override Switch
      | 0 = Use Model
      | 1 = Use Constant
  note: Override Switch Subsystem
  note: This subsystem is used to override the model value of a signal to a constant value
  In1 : Inport
  APP_Mismatch_Override : Constant  Value=Mismatch_APP_ON
  Constant : Constant  Value=0
  Multiport Switch : MultiPortSwitch  DataPortOrder=Zero-based contiguous  Inputs=2
  Out1 : Outport
  wires:
  Constant/1 -> Multiport Switch/3
  Multiport Switch/1 -> Out1/1
  In1/1 -> Multiport Switch/2
  APP_Mismatch_Override/1 -> Multiport Switch/1

== system Hybrid_P2_Parallel/Fault Trigger /Driver Interface Diagnostics setting/Override  BPP_Flt ==
  note: Signal Override Switch
      | 0 = Use Model
      | 1 = Use Constant
  note: This subsystem is used to override the model value of a signal to a constant value
  note: Override Switch Subsystem
  In1 : Inport
  Brk_Flt_ON : Constant  Value=Brk_Flt_ON
  Constant : Constant  Value=0
  Multiport Switch : MultiPortSwitch  DataPortOrder=Zero-based contiguous  Inputs=2
  Out1 : Outport
  wires:
  Brk_Flt_ON/1 -> Multiport Switch/1
  In1/1 -> Multiport Switch/2
  Multiport Switch/1 -> Out1/1
  Constant/1 -> Multiport Switch/3

== system Hybrid_P2_Parallel/Fault Trigger /Driver Interface Diagnostics setting/Override  KeyPos_Flt ==
  note: Signal Override Switch
      | 0 = Use Model
      | 1 = Use Constant
  note: Override Switch Subsystem
  note: This subsystem is used to override the model value of a signal to a constant value
  In1 : Inport
  Constant : Constant  Value=0
  KeyPos_Flt_ON : Constant  Value=KeyPos_Flt_ON
  Multiport Switch : MultiPortSwitch  DataPortOrder=Zero-based contiguous  Inputs=2
  Out1 : Outport
  wires:
  Constant/1 -> Multiport Switch/3
  Multiport Switch/1 -> Out1/1
  In1/1 -> Multiport Switch/2
  KeyPos_Flt_ON/1 -> Multiport Switch/1

== system Hybrid_P2_Parallel/Fault Trigger /Driver Interface Diagnostics setting/Override  PRNDL_Flt ==
  note: Signal Override Switch
      | 0 = Use Model
      | 1 = Use Constant
  note: This subsystem is used to override the model value of a signal to a constant value
  note: Override Switch Subsystem
  In1 : Inport
  Constant : Constant  Value=0
  Multiport Switch : MultiPortSwitch  DataPortOrder=Zero-based contiguous  Inputs=2
  PRNDL_Flt_ON : Constant  Value=PRNDL_Flt_ON
  Out1 : Outport
  wires:
  PRNDL_Flt_ON/1 -> Multiport Switch/1
  In1/1 -> Multiport Switch/2
  Multiport Switch/1 -> Out1/1
  Constant/1 -> Multiport Switch/3

== system Hybrid_P2_Parallel/Camaro Plant Model/Clutch2/Clutch Plant/ Actuator ==
  In1 : Inport
  Actuator Position to Clutch Engagement Pressure : Lookup_n-D  NumberOfTableDimensions=1  BreakpointsForDimension1=|  Table=|  InternalRulePriority=Speed  RndMeth=Simplest  InputSameDT=on
      BreakpointsForDimension1=|
      | [0
      | 100
      | 200
      | 300
      | 400
      | 500
      | 600
      | 700
      | 800
      | 900
      | 1000
      | 1100
      | 1200
      | 1300
      | 1400
      | 1500
      | 1600
      | 1700
      | 1800
      | 1900
      | 2000
      | 2100
      | 2200
      | 2300
      | 2400
      | 2500
      | 2600
      | 2700
      | 2800
      | 2900
      | 3000
      | 3100
      | 3200
      | 3300
      | 3400
      | 3500
      | 3600
      | 3700
      | 3800
      | 3900
      | 4000
      | 4100
      | 4200
      | 4300
      | 4400
      | 4500
      | 4600
      | 4700
      | 4800
      | 4900
      | 5000
      | 5100
      | 5200
      | 5300
      | 5400
      | 5500
      | 5600
      | 5700
      | 5800
      | 5900
      | 6000
      | 6100
      | 6200
      | 6300
      | 6400
      | 
      | ]
      Table=|
      | [892800
      | 892800
      | 892800
      | 833280
      | 773760
      | 714240
      | 654720
      | 595200
      | 535680
      | 476160
      | 416640
      | 357120
      | 297600
      | 238080
      | 178560
      | 119040
      | 59520
      | 0
      | 0
      | 0
      | 0
      | 0
      | 0
      | 0
      | 0
      | 0
      | 0
      | 0
      | 0
      | 0
      | 0
      | 0
      | 0
      | 0
      | 0
      | 0
      | 0
      | 0
      | 0
      | 0
      | 0
      | 0
      | 0
      | 0
      | 0
      | 0
      | 0
      | 0
      | 0
      | 0
      | 0
      | 0
      | 0
      | 0
      | 0
      | 0
      | 0
      | 0
      | 0
      | 0
      | 0
      | 0
      | 0
      | 0
      | 0
      | 
      | 
      | ]
  Bus Selector : BusSelector  OutputSignals=CY01_posCurr
  Clutch Engagement Pressure Command : Outport
  wires:
  Actuator Position to Clutch Engagement Pressure/1 -> Clutch Engagement Pressure Command/1
  Bus Selector/1 -> Actuator Position to Clutch Engagement Pressure/1  "<CY01_posCurr>"
  In1/1 -> Bus Selector/1

== system Hybrid_P2_Parallel/Camaro Plant Model/Clutch2/Clutch Plant/ Sensors  ==
  In1 : Inport
  Actuator Position to Actuator Pressure : Lookup_n-D  NumberOfTableDimensions=1  BreakpointsForDimension1=|  Table=|  InternalRulePriority=Speed  RndMeth=Simplest  InputSameDT=on
      BreakpointsForDimension1=|
      | [0
      | 300
      | 400
      | 500
      | 600
      | 700
      | 800
      | 900
      | 1000
      | 1100
      | 1200
      | 1300
      | 1400
      | 1500
      | 1600
      | 1700
      | 1800
      | 1900
      | 2000
      | 2100
      | 2200
      | 2300
      | 2400
      | 2500
      | 2600
      | 2700
      | 2800
      | 2900
      | 3000
      | 3100
      | 3200
      | 3300
      | 3400
      | 3500
      | 3600
      | 3700
      | 3800
      | 3900
      | 4000
      | 4100
      | 4200
      | 4300
      | 4400
      | 4500
      | 4600
      | 4650
      | ]
      Table=|
      | [0.4
      | 1.2
      | 2.6
      | 4
      | 5.6
      | 6.8
      | 8.6
      | 10.4
      | 12.2
      | 14
      | 15.8
      | 17.4
      | 18.8
      | 19.6
      | 20.2
      | 20
      | 19.8
      | 19.6
      | 19
      | 18.8
      | 18.4
      | 18
      | 17.8
      | 17.6
      | 17.4
      | 17.2
      | 17
      | 16.8
      | 16.6
      | 16.6
      | 16.6
      | 16.8
      | 17
      | 17.2
      | 17.4
      | 17.8
      | 18
      | 18.4
      | 18.6
      | 19
      | 19.4
      | 20.4
      | 21.2
      | 25.4
      | 36.4
      | 41
      | ]
  Bus Creator : BusCreator  Inputs=1
  Bus Selector : BusSelector  OutputSignals=CY01_posCurr
  Pressure : Outport
  wires:
  Bus Creator/1 -> Pressure/1
  In1/1 -> Bus Selector/1
  Bus Selector/1 -> Actuator Position to Actuator Pressure/1  "<CY01_posCurr>"
  Actuator Position to Actuator Pressure/1 -> Bus Creator/1  "CY01_pCurr"

== system Hybrid_P2_Parallel/Camaro Plant Model/Clutch2/Clutch Plant/Subsystem ==
  Engine Inertia Out : Inport
  Clutch Engagement Pressure : Inport  Port=2
  Clutch Inertia : Constant  Value=clt.plant.init.inertia
  Sum5 : Sum  Inputs=++|  SaturateOnIntegerOverflow=on  InputSameDT=on  OutDataTypeStr=Inherit: Same as first input
  Switch2 : Switch  Criteria=u2 > Threshold  SaturateOnIntegerOverflow=on  InputSameDT=on
  Motor Inertia In : Outport
  wires:
  Switch2/1 -> Motor Inertia In/1
  Engine Inertia Out/1 -> Sum5/2
  Sum5/1 -> Switch2/1
  Clutch Inertia/1 -> Switch2/3, Sum5/1
  Clutch Engagement Pressure/1 -> Switch2/2

== system Hybrid_P2_Parallel/Camaro Plant Model/Scopes/AxlTrq_to_EngTrq2/Ratio Filter ==
  Ratio : Inport
  Abs : Abs
  Compare To Zero : simulink/Logic and Bit Operations/Compare To Zero  relop===  OutDataTypeStr=boolean
  Constant : Constant  Value=cal.Time.TrnsOvrllEstTrqRatioSwitch
  Mature_Delay : EC2_libraries/Mature_Delay
      settings: SourceProductName=The database C:\Users\vrajm\AppData\Roaming\MathWorks\MATLAB\R2017b\slblocks_master.db is locked, or a table in the database is locked. (database is locked)
  Memory1 : Memory  InitialCondition=1
  Switch1 : Switch  Threshold=1
  Switch2 : Switch  Threshold=1
  Filtered_Ratio : Outport
  wires:
  Ratio/1 -> Compare To Zero/1, Abs/1
  Compare To Zero/1 -> Mature_Delay/1, Switch2/2
  Abs/1 -> Switch1/1, Switch2/3
  Switch1/1 -> Switch2/1
  Constant/1 -> Mature_Delay/2
  Mature_Delay/1 -> Switch1/2
  Memory1/1 -> Switch1/3
  Switch2/1 -> Filtered_Ratio/1, Memory1/1  "gear_ratio"

== system Hybrid_P2_Parallel/Camaro Plant Model/Scopes/AxlTrq_to_MtrTrq2/Ratio Filter ==
  Ratio : Inport
  Abs : Abs
  Compare To Zero : simulink/Logic and Bit Operations/Compare To Zero  relop===  OutDataTypeStr=boolean
  Constant : Constant  Value=cal.Time.TrnsOvrllEstTrqRatioSwitch
  Mature_Delay : EC2_libraries/Mature_Delay
      settings: SourceProductName=The database C:\Users\vrajm\AppData\Roaming\MathWorks\MATLAB\R2017b\slblocks_master.db is locked, or a table in the database is locked. (database is locked)
  Memory1 : Memory  InitialCondition=1
  Switch1 : Switch  Threshold=1
  Switch2 : Switch  Threshold=1
  Filtered_Ratio : Outport
  wires:
  Ratio/1 -> Compare To Zero/1, Abs/1
  Compare To Zero/1 -> Mature_Delay/1, Switch2/2
  Abs/1 -> Switch1/1, Switch2/3
  Switch1/1 -> Switch2/1
  Constant/1 -> Mature_Delay/2
  Mature_Delay/1 -> Switch1/2
  Memory1/1 -> Switch1/3
  Switch2/1 -> Filtered_Ratio/1, Memory1/1  "gear_ratio"

== system Hybrid_P2_Parallel/Controller/HSC/Camaro Fault Detection/Component Diagnostic ==
  note: Component Diagnostics
  note: Component Status Setting Rule
      | xxx_CompStatus could be 0, 1, 2 or 3
      | 0: component needs to be offline
      | 1: component needs torque plant to deliver creep torque
      | 2: component needs torque plant to limit maximum torque delivery
      | 3: component needs torque plant to operate normally
  SignalDiag : Inport
  Bus Creator : BusCreator  Inputs=6
  Driver Input Diagnostic : Subsystem
  ESS Component Diagnostic : Subsystem
  Engine Component Diagnostic : Subsystem
  Override Driver Status : Subsystem
  Override ESS Status : Subsystem
  Override Engine Status : Subsystem
  Override TCM Status : Subsystem
  Transmission Component Diagnostic : Subsystem
  CompDiag : Outport
  wires:
  Engine Component Diagnostic/2(Out2) -> Bus Creator/4  "EngTrqMismchType"
  Override Driver Status/1(Out1) -> Bus Creator/1  "Driver_Input_Status"
  Override TCM Status/1(Out1) -> Bus Creator/5  "TCM_Status"
  Override Engine Status/1(Out1) -> Bus Creator/3  "ECM_Status"
  Override ESS Status/1(Out1) -> Bus Creator/2  "BMS_Status"
  Transmission Component Diagnostic/1(Out1) -> Override TCM Status/1(In1)  "TCM_CompDiag"
  Engine Component Diagnostic/1(Out1) -> Override Engine Status/1(In1)  "ECM_CompDiag"
  ESS Component Diagnostic/1(Out1) -> Override ESS Status/1(In1)  "ESS_CompDiag"
  Driver Input Diagnostic/1(Out1) -> Override Driver Status/1(In1)  "Diver_CompDiag"
  Bus Creator/1 -> CompDiag/1
  SignalDiag/1 -> Driver Input Diagnostic/1(In1), ESS Component Diagnostic/1(In1), Bus Creator/6, Transmission Component Diagnostic/1(In1), Engine Component Diagnostic/1(In1)  "RawSig"

== system Hybrid_P2_Parallel/Controller/HSC/Camaro Fault Detection/Input Conversions ==
  note: These subsystems convert variable types to match those used in the
      | supervisor. In addition, override switches installed on each signal can
      | be used to manually override and signal for testing purposes
  note: Input Conversions and Override Switches
  RawSig : Inport
  BMS_Conversions : Subsystem
  Bus Creator : BusCreator  Inputs=5
  DriverInput_Conversions : Subsystem
  ECM_Conversions : Subsystem
  TCM_Conversions : Subsystem
  VehSig : Outport
  wires:
  TCM_Conversions/1(Out1) -> Bus Creator/4
  ECM_Conversions/1(Out1) -> Bus Creator/3
  RawSig/1 -> BMS_Conversions/1(In1), ECM_Conversions/1(In1), TCM_Conversions/1(In1), Bus Creator/5, DriverInput_Conversions/1(In1)  "RawSig"
  BMS_Conversions/1(Out1) -> Bus Creator/2
  Bus Creator/1 -> VehSig/1  "InputConvAndOvrd"
  DriverInput_Conversions/1(Out1) -> Bus Creator/1

== system Hybrid_P2_Parallel/Controller/HSC/Camaro Fault Detection/Signal Diagnostic ==
  note: Signal Diagnostics
  note: These subsystems evaluate each signal for proper value range and other checks
  VehSig : Inport
  Bus Creator : BusCreator  Inputs=5
  Driver Signal Diagnostic : Subsystem
  ESS Signal Diagnostic : Subsystem
  Engine Signal Diagnostic : Subsystem
  Subsystem1 : Subsystem
      mask Display: fprintf('Signal Naming Rule')
  Transmission Signal Diagnostic : Subsystem
  SignalDiag : Outport
  wires:
  Bus Creator/1 -> SignalDiag/1  "SignalDiag"
  Transmission Signal Diagnostic/1(Out2) -> Bus Creator/4  "Transmission_SigDiag"
  Engine Signal Diagnostic/1(Engine_SigDiag) -> Bus Creator/3  "Engine_SigDiag"
  ESS Signal Diagnostic/1(ESS_SigDiag) -> Bus Creator/2  "ESS_SigDiag"
  Driver Signal Diagnostic/1(Driver_SigDiag) -> Bus Creator/1  "Driver_SigDiag"
  VehSig/1 -> Transmission Signal Diagnostic/1(Sensors1), Bus Creator/5, Engine Signal Diagnostic/1(Sensors1), Driver Signal Diagnostic/1(Sensors1), ESS Signal Diagnostic/1(Sensors1)
